simulink model "N3_Test2"  (R2014b)
settings: Solver=ode3  SolverMode=SingleTasking  StartTime=0.0  StopTime=1e-2  FixedStep=fpgaclk  RelTol=1e-3
PreLoadFcn:
  | %fpgaclk=1/49.152e6
  | fpgaclk=1/49.152e6
  | 
  | SerialData=[1,zeros(1,11),1,0,0,1]
  | load ../../window
  | win=win';  %Go back to using flatter and wider windowed sync function
  | %load ../../hanning    %use Hahn window
  | 
  | load ../../PREemphasis   %For pre-empasis and deemphasis FIRs
  | 
  | %LUT3=xls2LUT2('../IQI_Qdemod.xls'); LUT3
  | load ../../LUT3
  | load ../../FIRiq2
  | % xls2LUT
  | 
  | GetProgFiles
  | 
  | PinAssignments    %Get Pin references for TE0722
  | 
  | 
  | 
  | 
  | 
  | %LCD
  | LCDdata=[LCD_D7,LCD_D6,LCD_D5,LCD_D4,LCD_D3,LCD_D2,LCD_D1,LCD_D0] %Note MSB...LSB!
  | LCDctrl=[LCD_E,LCD_RW,LCD_RS];
  | 
  | %for RS232 on pins 3 and 5 of USBB
  | 
  | %BT chip connections for WT12
  | 
  | RX_BT=RXD
  | TX_BT=TXD
  | 
  | RST_BB=RES
  | 
  | %PCMC=PCMC
  | %PCMS=PCMS
  | %PCMI=PCMI
  | %PCMO=PCMO
  | 
  | %Aliases:
  | SRDBT=PCMI
  | STDBT=PCMO
  | SCLK_BT=PCMC
  | SFS_BT=PCMS
  | 
  | %ADC control
  | 
  | %SDOA=SDOA
  | %SDOB=SDOB
  | %SCK=SCK
  | CONV=Csbar
  | CAL=Cal
  | 
  | ADC_G=[ADC_G3,ADC_G2,ADC_G1,ADC_G0]
  | %PD settings hard coded now
  | 
  | %%%%%%
  | TX_LOW=TX_Low
  | 
  | %Leds
  | %Defined inPinassignments
  | 
  | 
  | 
  | %TouchPads
  | %Defined in Pinassignments
  | 
  | 
  | 'Got to end of pre-load OK'
StartFcn:
  | fpgaclk=1/49.152e6
  | SerialData=[1,zeros(1,11),1,0,0,1]
values from neighbouring files (symbols this model uses):
  ADC_G0 = {'P10'}    [PinAssignments.m]
  ADC_G1 = {'P11'}    [PinAssignments.m]
  ADC_G2 = {'N14'}    [PinAssignments.m]
  ADC_G3 = {'M11'}    [PinAssignments.m]
  Cal = {'L12'}    [PinAssignments.m]
  Csbar = {'M12'}    [PinAssignments.m]
  LCD_D0 = {'J13'}    [PinAssignments.m]
  LCD_D1 = {'J14'}    [PinAssignments.m]
  LCD_D2 = {'F15'}    [PinAssignments.m]
  LCD_D3 = {'H14'}    [PinAssignments.m]
  LCD_D4 = {'G12'}    [PinAssignments.m]
  LCD_D5 = {'L15'}    [PinAssignments.m]
  LCD_D6 = {'M14'}    [PinAssignments.m]
  LCD_D7 = {'K15'}    [PinAssignments.m]
  PCMC = {'H11'}    [PinAssignments.m]
  PCMI = {'H12'}    [PinAssignments.m]
  PCMO = {'N13'}    [PinAssignments.m]
  PCMS = {'M10'}    [PinAssignments.m]
  RES = {'G11'}    [PinAssignments.m]
  RXD = {'H13'}    [PinAssignments.m]
  TX_Low = {'P15'}    [PinAssignments.m]
  TXD = {'P13'}    [PinAssignments.m]
undefined symbols (not defined in the file or in its folder): Down, Up
libraries: xbsIndex_r4 x126, MyFunctions x5
settings Model: Creator=Graham  LastModifiedBy=graham
settings DataIOCC: SignalLoggingSaveFormat=ModelDataLogs  SignalLoggingName=sigsOut
settings OptimizationCC: ExpressionDepthLimit=2147483647  InitFltsAndDblsToZero=on
settings DebuggingCC: SaveWithParameterizedLinksMsg=none  UnderspecifiedInitializationDetection=Classic  MergeDetectMultiDrivingBlocksExec=none  SignalResolutionControl=TryResolveAllWithWarning  SolverPrmCheckMsg=none  MultiTaskDSMMsg=warning  MultiTaskCondExecSysMsg=none  StateNameClashWarn=warning
settings HardwareCC: TargetUnknown=on
settings RTWCC: IncludeERTFirstTime=on
settings GRTTargetCC: TargetFcnLib=ansi_tfl_tmw.mat  ModelReferenceCompliant=off  CombineOutputUpdateFcns=off  MatFileLogging=off  GRTInterface=on

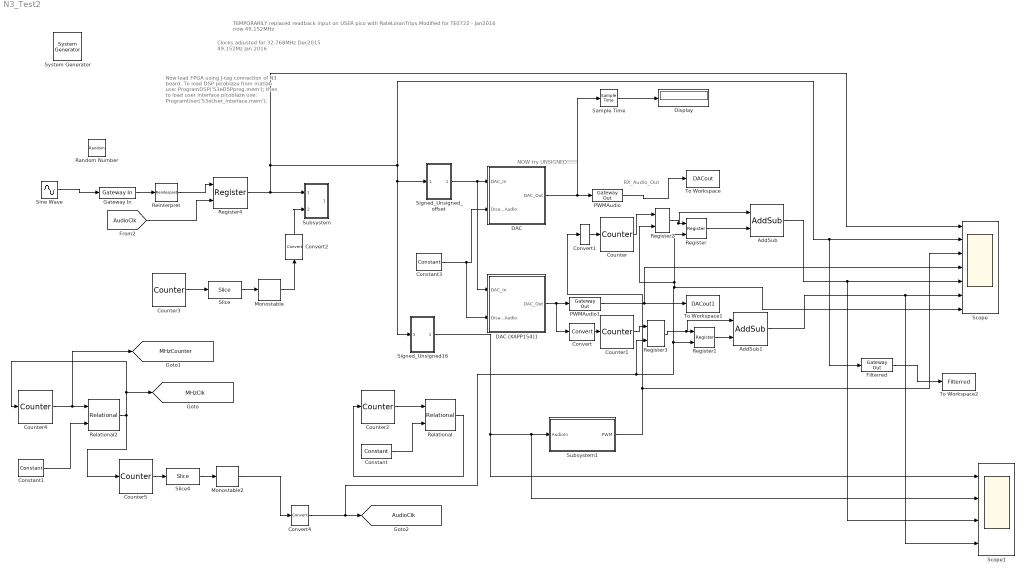
== system N3_Test2 ==
  note: RX_Audio_Out
  note: Now load FPGA using J-tag connection
      | of N3 board.
      | To load DSP picoblaze from matlab use:
      | ProgramDSP('S3eDSPprog.mem');
      | then to load user interface picoblaze use:
      | ProgramUser('S3eUser_interface.mem');
  note: Clocks adjusted for 32.768MHz Dec2015
      | 49.152Mz Jan 2016
  note: NOW try UNSIGNED!!!!!
  note: TEMPORARILY replaced readback input on USER pico with RateLoranTrips
      | Modified for TE0722 - Jan2016 now 49.152MHz
  " System Generator" : xbsIndex_r4/ System Generator  Tag=genX  xilinxfamily=zynq  part=xc7z010  speed=-1  package=clg225  synthesis_tool=XST  clock_wrapper=Clock Enables  directory=../../../SysgenOutput/TE0722  proj_type=Project Navigator  Synth_file=XST Defaults  Impl_file=ISE Defaults  testbench=off  simulink_period=fpgaclk  sysclk_period=30  dcm_input_clock_period=100  incr_netlist=off  trim_vbits=Everywhere in SubSystem  dbl_ovrd=According to Block Masks  core_generation=According to Block Masks  run_coregen=off  deprecated_control=off  eval_field=0  block_type=sysgen
      settings: block_version=8.2.02
  AddSub : xbsIndex_r4/AddSub  mode=Subtraction  use_carryin=off  use_carryout=off  en=off  latency=1  precision=Full  arith_type=Unsigned  n_bits=16  bin_pt=14  quantization=Truncate  overflow=Wrap  use_behavioral_HDL=off  hw_selection=Fabric  pipelined=off  dbl_ovrd=off  block_type=addsub
  AddSub1 : xbsIndex_r4/AddSub  mode=Subtraction  use_carryin=off  use_carryout=off  en=off  latency=1  precision=Full  arith_type=Unsigned  n_bits=16  bin_pt=14  quantization=Truncate  overflow=Wrap  use_behavioral_HDL=off  hw_selection=Fabric  pipelined=off  dbl_ovrd=off  block_type=addsub
  Constant : xbsIndex_r4/Constant  const=6142  gui_display_data_type=Fixed-point  arith_type=Unsigned  n_bits=13  bin_pt=0  preci_type=Single  exp_width=8  frac_width=24  explicit_period=off  period=1  equ=P=C  opselect=C  inp2=PCIN>>17  opr=+  inp1=P  carry=CIN  dbl_ovrd=off  block_type=constant
  Constant1 : xbsIndex_r4/Constant  const=46  gui_display_data_type=Fixed-point  arith_type=Unsigned  n_bits=6  bin_pt=0  preci_type=Single  exp_width=8  frac_width=24  explicit_period=on  period=fpgaclk  equ=P=C  opselect=C  inp2=PCIN>>17  opr=+  inp1=P  carry=CIN  dbl_ovrd=off  block_type=constant
      settings: block_version=VER_STRING_GOES_HERE
  Constant3 : xbsIndex_r4/Constant  const=0  gui_display_data_type=Boolean  arith_type=Boolean  n_bits=16  bin_pt=0  preci_type=Single  exp_width=8  frac_width=24  explicit_period=on  period=fpgaclk  equ=P=C  opselect=C  inp2=PCIN>>17  opr=+  inp1=P  carry=CIN  dbl_ovrd=off  block_type=constant
      settings: block_version=VER_STRING_GOES_HERE
  Convert{,1..2,4} (4 alike) : xbsIndex_r4/Convert  gui_display_data_type=Boolean  arith_type=Boolean  n_bits=16  bin_pt=14  float_type=Single  exp_bits=8  fraction_bits=24  quantization=Truncate  overflow=Wrap  en=off  latency=0  pipeline=off  dbl_ovrd=off  block_type=convert
  Counter : xbsIndex_r4/Counter  cnt_type=Free Running  cnt_to=Inf  operation=Up/Down  start_count=0  cnt_by_val=1  arith_type="Signed  (2's comp)"  n_bits=20  bin_pt=0  load_pin=off  rst=off  en=off  explicit_period=on  period=fpgaclk  use_behavioral_HDL=off  implementation=Fabric  dbl_ovrd=off  block_type=counter
  Counter1 : xbsIndex_r4/Counter  cnt_type=Free Running  cnt_to=Inf  operation=Up/Down  start_count=0  cnt_by_val=1  arith_type="Signed  (2's comp)"  n_bits=20  bin_pt=0  load_pin=off  rst=off  en=off  explicit_period=on  period=fpgaclk  use_behavioral_HDL=off  implementation=Fabric  dbl_ovrd=off  block_type=counter
  Counter2 : xbsIndex_r4/Counter  cnt_type=Free Running  cnt_to=Inf  operation=Up  start_count=0  cnt_by_val=1  arith_type=Unsigned  n_bits=13  bin_pt=0  load_pin=off  rst=on  en=off  explicit_period=on  period=fpgaclk  use_behavioral_HDL=off  implementation=Fabric  dbl_ovrd=off  block_type=counter
  Counter3 : xbsIndex_r4/Counter  cnt_type=Free Running  cnt_to=Inf  operation=Up  start_count=0  cnt_by_val=1  arith_type=Unsigned  n_bits=10  bin_pt=0  load_pin=off  rst=off  en=off  explicit_period=on  period=fpgaclk  use_behavioral_HDL=off  implementation=Fabric  dbl_ovrd=off  block_type=counter
  Counter4 : xbsIndex_r4/Counter  cnt_type=Free Running  cnt_to=Inf  operation=Up  start_count=0  cnt_by_val=1  arith_type=Unsigned  n_bits=6  bin_pt=0  load_pin=off  rst=on  en=off  explicit_period=on  period=fpgaclk  use_behavioral_HDL=off  implementation=Fabric  dbl_ovrd=off  block_type=counter
  Counter5 : xbsIndex_r4/Counter  cnt_type=Free Running  cnt_to=Inf  operation=Up  start_count=0  cnt_by_val=1  arith_type=Unsigned  n_bits=7  bin_pt=0  load_pin=off  rst=off  en=on  explicit_period=on  period=fpgaclk  use_behavioral_HDL=off  implementation=Fabric  dbl_ovrd=off  block_type=counter
  DAC : Subsystem
  DAC (XAPP154)1 : Subsystem
  Display : Display
  Filterred : xbsIndex_r4/Gateway Out  inherit_from_input=off  hdl_port=on  rows=1  columns=1  UseAsDAC=off  DACChannel='1'  interface=None  automatic_assignment=on  address_offset=hex2dec('00')  intf_description=''  timing_constraint=None  locs_specified=off  LOCs=PWMAudio  io_standard={'LVCMOS33'}  block_type=gatewayout
      settings: xl_area=[0, 0, 0, 0, 0, 0, 0]  block_version=VER_STRING_GOES_HERE
  Gateway In : xbsIndex_r4/Gateway In  gui_display_data_type=Fixed-point  arith_type="Signed  (2's comp)"  n_bits=16  bin_pt=15  preci_type=Single  exp_width=8  frac_width=24  rows=1  columns=1  quantization="Round  (unbiased: +/- Inf)"  overflow=Saturate  period=fpgaclk  UseAsADC=off  ADCChannel='1'  interface=None  automatic_assignment=on  address_offset=hex2dec('00')  intf_description=''  timing_constraint=None  locs_specified=off  LOCs={}  io_standard={}  inherit_from_input=off  hdl_port=on  dbl_ovrd=off  block_type=gatewayin
  Monostable : MyFunctions/Monostable
  Monostable2 : MyFunctions/Monostable
  PWMAudio : xbsIndex_r4/Gateway Out  inherit_from_input=off  hdl_port=on  rows=1  columns=1  UseAsDAC=off  DACChannel='1'  interface=None  automatic_assignment=on  address_offset=hex2dec('00')  intf_description=''  timing_constraint=None  locs_specified=on  LOCs=PWMAudio  io_standard={'LVCMOS33'}  block_type=gatewayout
      settings: xl_area=[0, 0, 0, 0, 0, 0, 0]  block_version=VER_STRING_GOES_HERE
  PWMAudio1 : xbsIndex_r4/Gateway Out  inherit_from_input=off  hdl_port=on  rows=1  columns=1  UseAsDAC=off  DACChannel='1'  interface=None  automatic_assignment=on  address_offset=hex2dec('00')  intf_description=''  timing_constraint=None  locs_specified=on  LOCs=PWMAudio  io_standard={'LVCMOS33'}  block_type=gatewayout
      settings: xl_area=[0, 0, 0, 0, 0, 0, 0]  block_version=VER_STRING_GOES_HERE
  Random Number : RandomNumber  Variance=0.002  SampleTime=fpgaclk*6144
  Register{,1..4} (5 alike) : xbsIndex_r4/Register  init=0  rst=off  en=on  dbl_ovrd=off  block_type=register
  Reinterpret : xbsIndex_r4/Reinterpret  force_arith_type=on  arith_type="Signed  (2's comp)"  force_bin_pt=on  bin_pt=0  block_type=cast
      settings: block_version=VER_STRING_GOES_HERE
  Relational : xbsIndex_r4/Relational  mode=a=b  op_type=Bool  en=off  latency=1  dbl_ovrd=off  block_type=relational
  Relational2 : xbsIndex_r4/Relational  mode=a=b  op_type=Bool  en=off  latency=1  dbl_ovrd=off  block_type=relational
  Sample Time : xbsIndex_r4/Sample Time  block_type=sampletime
      settings: infoedit="The Sample Time block reports the normalized sample period of its input.  A signal's normalized sample period is not equivalent to its Simulink absolute sample period.<br><br>Hardware notes: This block is implemented as a constant in hardware."
  Scope : Scope  NumInputPorts=7
      settings: YMin=-2500~-100~0~0~-50~-200~-5  YMax=3000~900~1~1~150~150~5
  Scope1 : Scope  NumInputPorts=4
      settings: YMin=-2500~-100~0~0  YMax=3000~900~1~1
  Signed_Unsigned16 : Subsystem
  Signed_Unsigned_offset : Subsystem
  Sine Wave : Sin  Amplitude=0.9  Frequency=6.3e2  SampleTime=0
  Slice : xbsIndex_r4/Slice  nbits=1  boolean_output=off  mode=Upper Bit Location + Width  bit1=0  base1=MSB of Input  bit0=0  base0=LSB of Input  dbl_ovrd=off  block_type=slice
  Slice4 : xbsIndex_r4/Slice  nbits=1  boolean_output=off  mode=Upper Bit Location + Width  bit1=0  base1=MSB of Input  bit0=0  base0=LSB of Input  dbl_ovrd=off  block_type=slice
  Subsystem : Subsystem
  Subsystem1 : Subsystem
  To Workspace : ToWorkspace  VariableName=DACout  SampleTime=-1
  To Workspace1 : ToWorkspace  VariableName=DACout1  SampleTime=-1
  To Workspace2 : ToWorkspace  VariableName=Filterred  SampleTime=-1
  tag scope: AudioClk=global, MHzClk=global, MHzCounter=global
  wires:
  PWMAudio/1 -> To Workspace/1
  DAC/1(DAC_Out) -> Sample Time/1, PWMAudio/1
  Signed_Unsigned_offset/1(Out1) -> DAC (XAPP154)1/1(DAC_In), DAC/1(DAC_In)
  Constant3/1 -> DAC (XAPP154)1/2(Disable_Audio), DAC/2(Disable_Audio)
  DAC (XAPP154)1/1(DAC_Out) -> Convert/1, PWMAudio1/1
  Gateway In/1 -> Reinterpret/1
  PWMAudio1/1 -> Scope/4, To Workspace1/1
  Sample Time/1 -> Display/1
  Convert/1 -> Counter1/1
  Convert1/1 -> Counter/1
  Counter2/1 -> Relational/1
  Constant/1 -> Relational/2
  Convert4/1 -> Register3/2, Register1/2, Scope/7, Register2/2, Register/2, [AudioClk]
  Counter/1 -> Register2/1
  Register/1 -> AddSub/2
  AddSub/1 -> Scope1/3, Scope/5
  Counter1/1 -> Register3/1
  Register1/1 -> AddSub1/2
  AddSub1/1 -> Scope1/4, Scope/6
  Register2/1 -> AddSub/1, Register/1
  Register3/1 -> AddSub1/1, Register1/1
  Reinterpret/1 -> Register4/1
  Slice/1 -> Monostable/1
  Counter3/1 -> Slice/1
  Monostable/1 -> Convert2/1
  Convert2/1 -> Subsystem/2(In3)
  Filterred/1 -> To Workspace2/1
  Counter4/1 -> [MHzCounter], Relational2/1
  Constant1/1 -> Relational2/2
  Relational2/1 -> Counter5/1, [MHzClk], Counter4/1
  Slice4/1 -> Monostable2/1
  Counter5/1 -> Slice4/1
  Monostable2/1 -> Convert4/1
  Subsystem1/1(PWM) -> Scope/3, Convert1/1
  Signed_Unsigned16/1(Out1) -> Scope1/1, Scope1/2, Subsystem1/1(AudioIn)
  Sine Wave/1 -> Gateway In/1
  Register4/1 -> Signed_Unsigned16/1(In1), Signed_Unsigned_offset/1(In1), Filterred/1, Scope/2, Scope/1, Subsystem/1(In1)
  [AudioClk] -> Register4/2
  Relational/1 -> Counter2/1

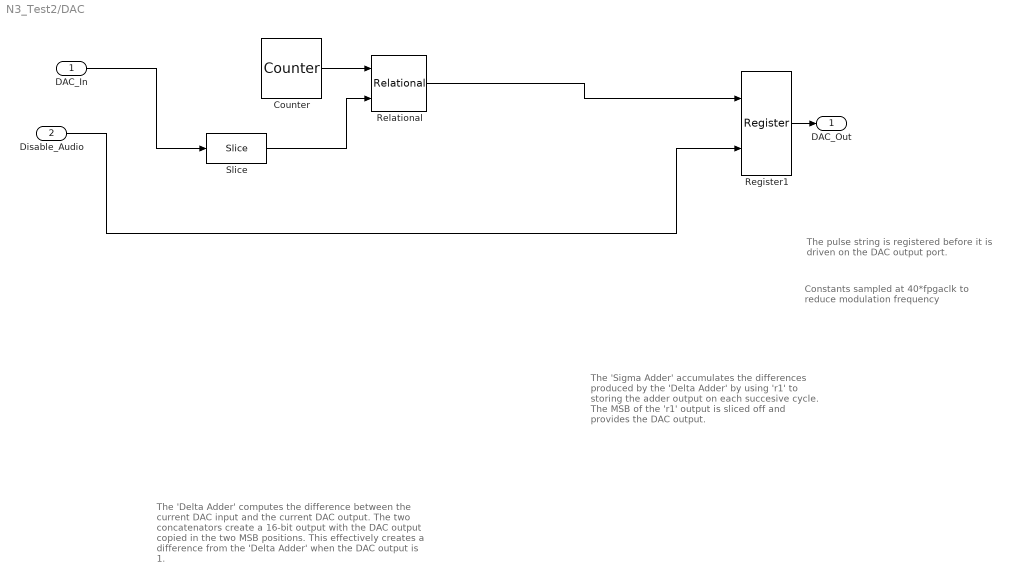
== system N3_Test2/DAC ==
  note: The 'Delta Adder' computes the difference
      | between the current DAC input and the current
      | DAC output.  The two concatenators create
      | a 16-bit output with the DAC output copied in the
      | two MSB positions. This effectively creates a
      | difference from the 'Delta Adder' when the DAC
      | output is 1.
  note: The 'Sigma Adder' accumulates the
      | differences produced by the 'Delta Adder'
      | by using 'r1' to storing the adder output on
      | each succesive cycle.  The MSB of the 'r1'
      | output is sliced off and provides the DAC
      | output.
  note: The pulse string is registered before
      | it is driven on the DAC output port.
  note: Constants sampled at 40*fpgaclk
      | to reduce modulation frequency
  DAC_In : Inport
  Disable_Audio : Inport  Port=2
  Counter : xbsIndex_r4/Counter  cnt_type=Free Running  cnt_to=Inf  operation=Up  start_count=0  cnt_by_val=1  arith_type=Unsigned  n_bits=8  bin_pt=0  load_pin=off  rst=off  en=off  explicit_period=on  period=fpgaclk  use_behavioral_HDL=off  implementation=Fabric  dbl_ovrd=off  block_type=counter
  Register1 : xbsIndex_r4/Register  init=0  rst=on  en=off  dbl_ovrd=off  block_type=register
      settings: xl_area=[1 1 0 0 0 0 0]  block_version=VER_STRING_GOES_HERE
  Relational : xbsIndex_r4/Relational  mode=a<b  op_type=Bool  en=off  latency=1  dbl_ovrd=off  block_type=relational
  Slice : xbsIndex_r4/Slice  nbits=8  boolean_output=off  mode=Upper Bit Location + Width  bit1=0  base1=MSB of Input  bit0=0  base0=LSB of Input  dbl_ovrd=off  block_type=slice
  DAC_Out : Outport
  wires:
  Register1/1 -> DAC_Out/1
  Disable_Audio/1 -> Register1/2
  DAC_In/1 -> Slice/1
  Counter/1 -> Relational/1
  Slice/1 -> Relational/2
  Relational/1 -> Register1/1

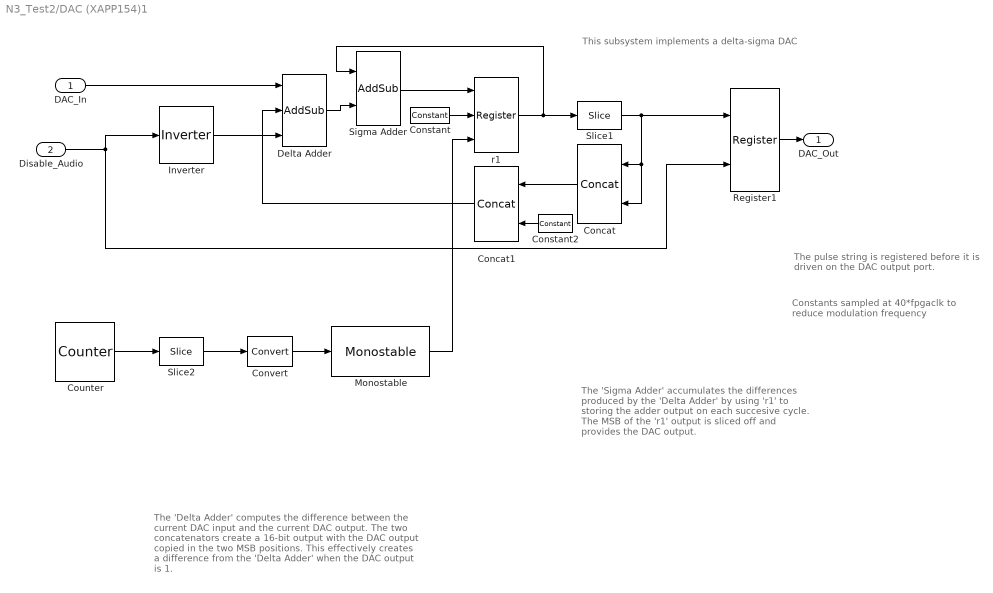
== system N3_Test2/DAC (XAPP154)1 ==
  note: This subsystem implements a delta-sigma DAC
  note: The 'Delta Adder' computes the difference
      | between the current DAC input and the current
      | DAC output.  The two concatenators create
      | a 16-bit output with the DAC output copied in the
      | two MSB positions. This effectively creates a
      | difference from the 'Delta Adder' when the DAC
      | output is 1.
  note: The 'Sigma Adder' accumulates the
      | differences produced by the 'Delta Adder'
      | by using 'r1' to storing the adder output on
      | each succesive cycle.  The MSB of the 'r1'
      | output is sliced off and provides the DAC
      | output.
  note: The pulse string is registered before
      | it is driven on the DAC output port.
  note: Constants sampled at 40*fpgaclk
      | to reduce modulation frequency
  DAC_In : Inport
  Disable_Audio : Inport  Port=2
  Concat : xbsIndex_r4/Concat  num_inputs=2  dbl_ovrd=off  block_type=concat
      settings: block_version=VER_STRING_GOES_HERE
  Concat1 : xbsIndex_r4/Concat  num_inputs=2  dbl_ovrd=off  block_type=concat
      settings: block_version=VER_STRING_GOES_HERE
  Constant : xbsIndex_r4/Constant  const=0  gui_display_data_type=Boolean  arith_type=Boolean  n_bits=1  bin_pt=0  preci_type=Single  exp_width=8  frac_width=24  explicit_period=on  period=fpgaclk  equ=P=C  opselect=C  inp2=PCIN>>17  opr=+  inp1=P  carry=CIN  dbl_ovrd=off  block_type=constant
      settings: block_version=VER_STRING_GOES_HERE
  Constant2 : xbsIndex_r4/Constant  const=0  gui_display_data_type=Fixed-point  arith_type=Unsigned  n_bits=14  bin_pt=0  preci_type=Single  exp_width=8  frac_width=24  explicit_period=on  period=fpgaclk  equ=P=C  opselect=C  inp2=PCIN>>17  opr=+  inp1=P  carry=CIN  dbl_ovrd=off  block_type=constant
      settings: block_version=VER_STRING_GOES_HERE
  Convert : xbsIndex_r4/Convert  gui_display_data_type=Boolean  arith_type=Boolean  n_bits=16  bin_pt=14  float_type=Single  exp_bits=8  fraction_bits=24  quantization=Truncate  overflow=Wrap  en=off  latency=0  pipeline=off  dbl_ovrd=off  block_type=convert
  Counter : xbsIndex_r4/Counter  cnt_type=Free Running  cnt_to=Inf  operation=Up  start_count=0  cnt_by_val=1  arith_type=Unsigned  n_bits=6  bin_pt=0  load_pin=off  rst=off  en=off  explicit_period=on  period=fpgaclk  use_behavioral_HDL=off  implementation=Fabric  dbl_ovrd=off  block_type=counter
  Delta Adder : xbsIndex_r4/AddSub  mode=Addition  use_carryin=off  use_carryout=off  en=on  latency=1  precision=User Defined  arith_type=Unsigned  n_bits=16  bin_pt=0  quantization=Truncate  overflow=Wrap  use_behavioral_HDL=on  hw_selection=Fabric  pipelined=off  use_rpm=off  dbl_ovrd=off  block_type=addsub
      settings: xl_area=[8 0 0 16 0 0 0]  block_version=VER_STRING_GOES_HERE
  Inverter : xbsIndex_r4/Inverter  en=off  latency=0  dbl_ovrd=off  block_type=inv
      settings: block_version=8.2.02
  Monostable : MyFunctions/Monostable
  Register1 : xbsIndex_r4/Register  init=0  rst=on  en=off  dbl_ovrd=off  block_type=register
      settings: xl_area=[1 1 0 0 0 0 0]  block_version=VER_STRING_GOES_HERE
  Sigma Adder : xbsIndex_r4/AddSub  mode=Addition  use_carryin=off  use_carryout=off  en=off  latency=0  precision=User Defined  arith_type=Unsigned  n_bits=16  bin_pt=0  quantization=Truncate  overflow=Wrap  use_behavioral_HDL=on  hw_selection=Fabric  pipelined=off  use_rpm=off  dbl_ovrd=off  block_type=addsub
      settings: xl_area=[8 0 0 16 0 0 0]  block_version=VER_STRING_GOES_HERE
  Slice1 : xbsIndex_r4/Slice  nbits=1  boolean_output=off  mode=Upper Bit Location + Width  bit1=0  base1=MSB of Input  bit0=0  base0=LSB of Input  dbl_ovrd=off  block_type=slice
      settings: infoedit="Extracts a given range of bits from each input sample and presents it at the output.  The output type is ordinarily unsigned with binary point at zero, but can be Boolean when the slice is one bit wide.<P><P>Hardware notes: In hardware this block costs nothing."  block_version=VER_STRING_GOES_HERE
  Slice2 : xbsIndex_r4/Slice  nbits=1  boolean_output=off  mode=Upper Bit Location + Width  bit1=0  base1=MSB of Input  bit0=0  base0=LSB of Input  dbl_ovrd=off  block_type=slice
      settings: block_version=VER_STRING_GOES_HERE
  r1 : xbsIndex_r4/Register  init=2^6  rst=on  en=on  dbl_ovrd=off  block_type=register
      settings: xl_area=[8 16 0 0 0 0 0]  block_version=VER_STRING_GOES_HERE
  DAC_Out : Outport
  wires:
  DAC_In/1 -> Delta Adder/1
  Register1/1 -> DAC_Out/1
  r1/1 -> Slice1/1, Sigma Adder/1
  Sigma Adder/1 -> r1/1
  Constant/1 -> r1/2
  Concat1/1 -> Delta Adder/2
  Concat/1 -> Concat1/1
  Slice1/1 -> Register1/1, Concat/1, Concat/2
  Constant2/1 -> Concat1/2
  Delta Adder/1 -> Sigma Adder/2
  Disable_Audio/1 -> Register1/2, Inverter/1
  Inverter/1 -> Delta Adder/3
  Counter/1 -> Slice2/1
  Slice2/1 -> Convert/1
  Monostable/1 -> r1/3
  Convert/1 -> Monostable/1

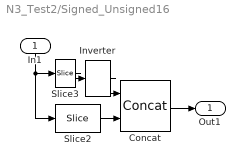
== system N3_Test2/Signed_Unsigned16 ==
  In1 : Inport
  Concat : xbsIndex_r4/Concat  num_inputs=2  dbl_ovrd=off  block_type=concat
      settings: block_version=VER_STRING_GOES_HERE
  Inverter : xbsIndex_r4/Inverter  en=off  latency=0  dbl_ovrd=off  block_type=inv
      settings: xl_area=[0, 0, 0, 0, 0, 0, 0]  block_version=VER_STRING_GOES_HERE
  Slice2 : xbsIndex_r4/Slice  nbits=15  boolean_output=off  mode=Upper Bit Location + Width  bit1=-1  base1=MSB of Input  bit0=0  base0=LSB of Input  dbl_ovrd=off  block_type=slice
      settings: block_version=VER_STRING_GOES_HERE
  Slice3 : xbsIndex_r4/Slice  nbits=1  boolean_output=off  mode=Upper Bit Location + Width  bit1=0  base1=MSB of Input  bit0=0  base0=LSB of Input  dbl_ovrd=off  block_type=slice
      settings: block_version=VER_STRING_GOES_HERE
  Out1 : Outport
  wires:
  Slice2/1 -> Concat/2
  Slice3/1 -> Inverter/1
  Inverter/1 -> Concat/1
  In1/1 -> Slice2/1, Slice3/1
  Concat/1 -> Out1/1

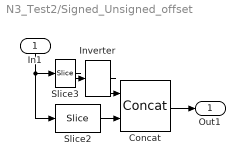
== system N3_Test2/Signed_Unsigned_offset ==
  In1 : Inport
  Concat : xbsIndex_r4/Concat  num_inputs=2  dbl_ovrd=off  block_type=concat
      settings: block_version=VER_STRING_GOES_HERE
  Inverter : xbsIndex_r4/Inverter  en=off  latency=0  dbl_ovrd=off  block_type=inv
      settings: xl_area=[0, 0, 0, 0, 0, 0, 0]  block_version=VER_STRING_GOES_HERE
  Slice2 : xbsIndex_r4/Slice  nbits=13  boolean_output=off  mode=Upper Bit Location + Width  bit1=-1  base1=MSB of Input  bit0=0  base0=LSB of Input  dbl_ovrd=off  block_type=slice
      settings: block_version=VER_STRING_GOES_HERE
  Slice3 : xbsIndex_r4/Slice  nbits=1  boolean_output=off  mode=Upper Bit Location + Width  bit1=0  base1=MSB of Input  bit0=0  base0=LSB of Input  dbl_ovrd=off  block_type=slice
      settings: block_version=VER_STRING_GOES_HERE
  Out1 : Outport
  wires:
  Slice2/1 -> Concat/2
  Slice3/1 -> Inverter/1
  Inverter/1 -> Concat/1
  In1/1 -> Slice2/1, Slice3/1
  Concat/1 -> Out1/1

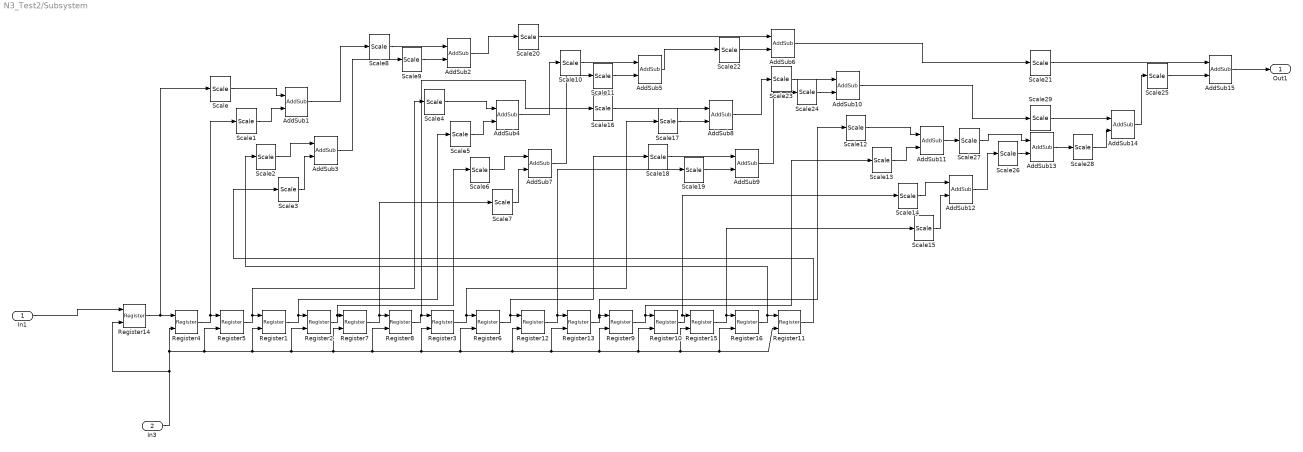
== system N3_Test2/Subsystem ==
  In1 : Inport
  In3 : Inport  Port=2
  AddSub{1..15} (15 alike) : xbsIndex_r4/AddSub  mode=Addition  use_carryin=off  use_carryout=off  en=off  latency=1  precision=User Defined  arith_type="Signed  (2's comp)"  n_bits=16  bin_pt=0  quantization=Truncate  overflow=Flag as error  use_behavioral_HDL=off  hw_selection=Fabric  pipelined=off  dbl_ovrd=off  block_type=addsub
  Register{1..16} (16 alike) : xbsIndex_r4/Register  init=0  rst=off  en=on  dbl_ovrd=off  block_type=register
  Scale{,1..3,21,28} (6 alike) : xbsIndex_r4/Scale  scale_factor=-2  dbl_ovrd=off  block_type=scale
  Scale{4..20,22..27,29} (24 alike) : xbsIndex_r4/Scale  scale_factor=-1  dbl_ovrd=off  block_type=scale
  Out1 : Outport
  wires:
  Register4/1 -> Scale1/1, Register5/1
  Register1/1 -> Scale5/1, Register2/1
  Register5/1 -> Scale4/1, Register1/1
  Register7/1 -> Scale7/1, Register8/1
  Register3/1 -> Scale17/1, Register6/1
  Register8/1 -> Scale16/1, Register3/1
  Register2/1 -> Scale6/1, Register7/1
  Register12/1 -> Scale19/1, Register13/1
  Register9/1 -> Scale13/1, Register10/1
  Register13/1 -> Scale12/1, Register9/1
  Register15/1 -> Scale15/1, Register16/1
  Register11/1 -> Scale3/1
  In3/1 -> Register14/2, Register7/2, Register12/2, Register15/2, Register11/2, Register16/2, Register10/2, Register9/2, Register13/2, Register6/2, Register3/2, Register8/2, Register2/2, Register1/2, Register5/2, Register4/2
  Register16/1 -> Scale2/1, Register11/1
  Register10/1 -> Scale14/1, Register15/1
  Register6/1 -> Scale18/1, Register12/1
  Scale1/1 -> AddSub1/2
  Scale/1 -> AddSub1/1
  Scale3/1 -> AddSub3/2
  Scale2/1 -> AddSub3/1
  AddSub3/1 -> Scale9/1
  AddSub1/1 -> Scale8/1
  Scale5/1 -> AddSub4/2
  Scale4/1 -> AddSub4/1
  Scale7/1 -> AddSub7/2
  Scale6/1 -> AddSub7/1
  AddSub7/1 -> Scale11/1
  AddSub4/1 -> Scale10/1
  AddSub9/1 -> Scale24/1
  AddSub8/1 -> Scale23/1
  Scale13/1 -> AddSub11/2
  Scale12/1 -> AddSub11/1
  Scale15/1 -> AddSub12/2
  Scale14/1 -> AddSub12/1
  AddSub12/1 -> Scale26/1
  AddSub11/1 -> Scale27/1
  AddSub2/1 -> Scale20/1
  AddSub5/1 -> Scale22/1
  AddSub10/1 -> Scale29/1
  AddSub13/1 -> Scale28/1
  AddSub6/1 -> Scale21/1
  AddSub14/1 -> Scale25/1
  AddSub15/1 -> Out1/1
  Scale8/1 -> AddSub2/1
  Scale9/1 -> AddSub2/2
  Scale10/1 -> AddSub5/1
  Scale11/1 -> AddSub5/2
  Scale16/1 -> AddSub8/1
  Scale17/1 -> AddSub8/2
  Scale18/1 -> AddSub9/1
  Scale19/1 -> AddSub9/2
  Scale20/1 -> AddSub6/1
  Scale21/1 -> AddSub15/1
  Scale22/1 -> AddSub6/2
  Scale23/1 -> AddSub10/1
  Scale24/1 -> AddSub10/2
  Scale25/1 -> AddSub15/2
  Scale26/1 -> AddSub13/2
  Scale27/1 -> AddSub13/1
  Scale28/1 -> AddSub14/2
  In1/1 -> Register14/1
  Register14/1 -> Scale/1, Register4/1
  Scale29/1 -> AddSub14/1

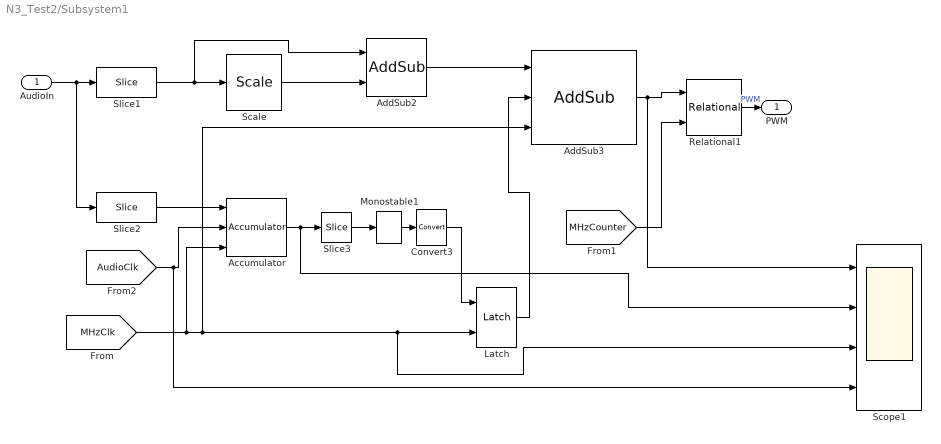
== system N3_Test2/Subsystem1 ==
  AudioIn : Inport
  Accumulator : xbsIndex_r4/Accumulator  operation=Add  n_bits=8  overflow=Wrap  scale=1  rst=on  hasbypass=off  infoeditControl=reset for floating point data type must be asserted for a minimum of 2 cycles  en=on  latency=1  msb_inp=100  msb=100  lsb=-100  use_behavioral_HDL=on  implementation=Fabric  dbl_ovrd=off  block_type=accum
  AddSub2 : xbsIndex_r4/AddSub  mode=Addition  use_carryin=off  use_carryout=off  en=off  latency=1  precision=User Defined  arith_type=Unsigned  n_bits=6  bin_pt=0  quantization=Truncate  overflow=Wrap  use_behavioral_HDL=off  hw_selection=Fabric  pipelined=off  dbl_ovrd=off  block_type=addsub
  AddSub3 : xbsIndex_r4/AddSub  mode=Addition  use_carryin=off  use_carryout=off  en=on  latency=1  precision=User Defined  arith_type=Unsigned  n_bits=6  bin_pt=0  quantization=Truncate  overflow=Wrap  use_behavioral_HDL=off  hw_selection=Fabric  pipelined=off  dbl_ovrd=off  block_type=addsub
  Convert3 : xbsIndex_r4/Convert  gui_display_data_type=Boolean  arith_type=Boolean  n_bits=16  bin_pt=14  float_type=Single  exp_bits=8  fraction_bits=24  quantization=Truncate  overflow=Wrap  en=off  latency=0  pipeline=off  dbl_ovrd=off  block_type=convert
  Latch : MyFunctions/Latch
      link override Set1: const=1  gui_display_data_type=Fixed-point  arith_type=Unsigned  n_bits=1  bin_pt=0  preci_type=Single  exp_width=8  frac_width=24  explicit_period=on  period=fpgaclk  equ=P=C  opselect=C  inp2=PCIN>>17  opr=+  inp1=P  carry=CIN  dbl_ovrd=off
  Monostable1 : MyFunctions/Monostable
  Relational1 : xbsIndex_r4/Relational  mode=a>b  op_type=Bool  en=off  latency=1  dbl_ovrd=off  block_type=relational
  Scale : xbsIndex_r4/Scale  scale_factor=-1  dbl_ovrd=off  block_type=scale
  Scope1 : Scope  NumInputPorts=4
      settings: YMin=-2500~-100~0~0  YMax=3000~900~1~1  SaveName=ScopeData2
  Slice1 : xbsIndex_r4/Slice  nbits=5  boolean_output=off  mode=Upper Bit Location + Width  bit1=0  base1=MSB of Input  bit0=0  base0=LSB of Input  dbl_ovrd=off  block_type=slice
  Slice2 : xbsIndex_r4/Slice  nbits=8  boolean_output=off  mode=Upper Bit Location + Width  bit1=-5  base1=MSB of Input  bit0=0  base0=LSB of Input  dbl_ovrd=off  block_type=slice
  Slice3 : xbsIndex_r4/Slice  nbits=1  boolean_output=off  mode=Upper Bit Location + Width  bit1=0  base1=MSB of Input  bit0=0  base0=LSB of Input  dbl_ovrd=off  block_type=slice
  PWM : Outport
  wires:
  Relational1/1 -> PWM/1  "PWM"
  Slice2/1 -> Accumulator/1
  Accumulator/1 -> Scope1/2, Slice3/1
  AudioIn/1 -> Slice2/1, Slice1/1
  Slice1/1 -> AddSub2/1, Scale/1
  Scale/1 -> AddSub2/2
  AddSub2/1 -> AddSub3/1
  Slice3/1 -> Monostable1/1
  Monostable1/1 -> Convert3/1
  Latch/1 -> AddSub3/2
  AddSub3/1 -> Scope1/1, Relational1/1
  [MHzClk] -> Scope1/3, Latch/2, AddSub3/3, Accumulator/3
  [MHzCounter] -> Relational1/2
  [AudioClk] -> Scope1/4, Accumulator/2
  Convert3/1 -> Latch/1
